simulink model "ScaledMotor"  (R2015a)
settings: Solver=ode45  StartTime=0.0  StopTime=10.0  RelTol=1e-3
settings Model: Creator=Justin  LastModifiedBy=Justin

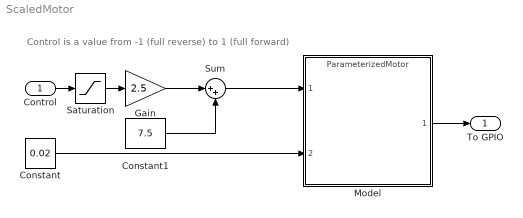
== system ScaledMotor ==
  note: Control is a value from -1 (full reverse) to 1 (full forward)
  Control : Inport
  Constant : Constant  Value=0.02
  Constant1 : Constant  Value=7.5
  Gain : Gain  Gain=2.5
  Model : ModelReference  ModelNameDialog=ParameterizedMotor.slx  SimulationMode=Normal  ModelReferenceVersion=1.11  CopyOfModelName=ParameterizedMotor.slx  DefaultDataLogging=on
  Saturation : Saturate  UpperLimit=1  LowerLimit=-1
  Sum : Sum  Inputs=|++
  To GPIO : Outport
  wires:
  Constant/1 -> Model/2
  Model/1 -> To GPIO/1
  Control/1 -> Saturation/1
  Saturation/1 -> Gain/1
  Gain/1 -> Sum/1
  Constant1/1 -> Sum/2
  Sum/1 -> Model/1
